simulink model "exo2_Part1_y"  (R2020b)
settings: Solver=VariableStepAuto  StartTime=0.0  StopTime=30  RelTol=1e-3
undefined symbols (not defined in the file or in its folder): fdesignblkfcn, gcbh
libraries: dspfdesign x4, vrlib x1
settings Model: Creator=aayush  LastModifiedBy=YNS
settings DebuggingCC: UnconnectedInputMsg=none  UnconnectedOutputMsg=none  UnconnectedLineMsg=none
settings ModelReferenceCC: EnableRefExpFcnMdlSchedulingChecks=off

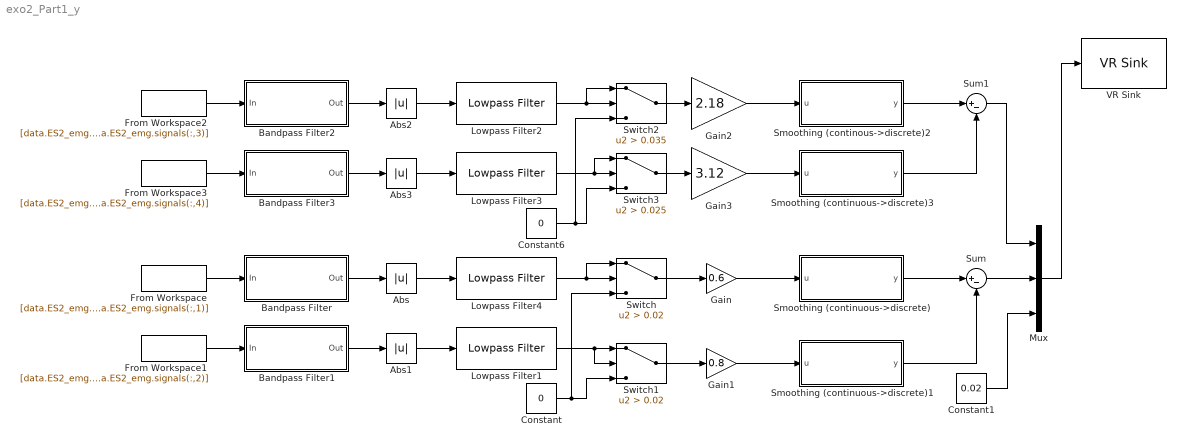
== system exo2_Part1_y ==
  Abs{,1..3} (4 alike) : Abs
  Bandpass Filter : Subsystem  DialogController=fdesignblkfcn  InitFcn=fdesignblkfcn(gcbh, {'InitFcn'});  mask(Bandpass Filter){}
      mask help: Design a bandpass filter
      settings: CopyFcn=fdesignblkfcn(gcbh, {'CopyFcn'});
      mask Help: helpview(mapfilelocation('dsp'), 'dspbandpassfilter');
      mask Display: disp('Bandpass');
  Bandpass Filter1 : Subsystem  DialogController=fdesignblkfcn  InitFcn=fdesignblkfcn(gcbh, {'InitFcn'});  mask(Bandpass Filter){}
      mask help: Design a bandpass filter
      settings: CopyFcn=fdesignblkfcn(gcbh, {'CopyFcn'});
      mask Help: helpview(mapfilelocation('dsp'), 'dspbandpassfilter');
      mask Display: disp('Bandpass');
  Bandpass Filter2 : Subsystem  DialogController=fdesignblkfcn  InitFcn=fdesignblkfcn(gcbh, {'InitFcn'});  mask(Bandpass Filter){}
      mask help: Design a bandpass filter
      settings: CopyFcn=fdesignblkfcn(gcbh, {'CopyFcn'});
      mask Help: helpview(mapfilelocation('dsp'), 'dspbandpassfilter');
      mask Display: disp('Bandpass');
  Bandpass Filter3 : Subsystem  DialogController=fdesignblkfcn  InitFcn=fdesignblkfcn(gcbh, {'InitFcn'});  mask(Bandpass Filter){}
      mask help: Design a bandpass filter
      settings: CopyFcn=fdesignblkfcn(gcbh, {'CopyFcn'});
      mask Help: helpview(mapfilelocation('dsp'), 'dspbandpassfilter');
      mask Display: disp('Bandpass');
  Constant : Constant  Value=0
  Constant1 : Constant  Value=0.02
  Constant6 : Constant  Value=0
  From Workspace : FromWorkspace  VariableName=[data.ES2_emg.time,data.ES2_emg.signals(:,1)]  SampleTime=1/3000
  From Workspace1 : FromWorkspace  VariableName=[data.ES2_emg.time,data.ES2_emg.signals(:,2)]  SampleTime=1/3000
  From Workspace2 : FromWorkspace  VariableName=[data.ES2_emg.time,data.ES2_emg.signals(:,3)]  SampleTime=1/3000
  From Workspace3 : FromWorkspace  VariableName=[data.ES2_emg.time,data.ES2_emg.signals(:,4)]  SampleTime=1/3000
  Gain : Gain  Gain=0.6
  Gain1 : Gain  Gain=0.8
  Gain2 : Gain  Gain=2.18
  Gain3 : Gain  Gain=3.12
  Lowpass Filter{1..4} (4 alike) : dspfdesign/Lowpass Filter  FilterType=FIR  DesignForMinimumOrder=on  FilterOrder=50  PassbandFrequency=3  StopbandFrequency=6  PassbandRipple=0.1  StopbandAttenuation=80  InheritSampleRate=off  SampleRate=1000  SimulateUsing=Interpreted execution  roundingMode=Floor  coeffsDataTypeStr=fixdt(1,16)
  Mux : Mux  Inputs=3
  Smoothing (continous->discrete)2 : Subsystem  mask(Smoothing (continuous->discrete)){tsSmoothing=0.35, smoothing0=0}
      mask prompts: tsSmoothing "physmod:simscape:couplers:SimscapeNetworkCouplersLib:SmoothingTimeConstants_MP"; smoothing0 "physmod:simscape:couplers:SimscapeNetworkCouplersLib:InitialOutput_MP"
      mask help: physmod:simscape:couplers:SimscapeNetworkCouplersLib:Smoothingcontinuousdiscrete_MD
      mask Help: web([docroot '/physmod/simscape/ref/networkcouplersmoothingcontinuousdiscrete.html'])
  Smoothing (continuous->discrete) : Subsystem  mask(Smoothing (continuous->discrete)){tsSmoothing=0.35, smoothing0=0}
      mask prompts: tsSmoothing "physmod:simscape:couplers:SimscapeNetworkCouplersLib:SmoothingTimeConstants_MP"; smoothing0 "physmod:simscape:couplers:SimscapeNetworkCouplersLib:InitialOutput_MP"
      mask help: physmod:simscape:couplers:SimscapeNetworkCouplersLib:Smoothingcontinuousdiscrete_MD
      mask Help: web([docroot '/physmod/simscape/ref/networkcouplersmoothingcontinuousdiscrete.html'])
  Smoothing (continuous->discrete)1 : Subsystem  mask(Smoothing (continuous->discrete)){tsSmoothing=0.35, smoothing0=0}
      mask prompts: tsSmoothing "physmod:simscape:couplers:SimscapeNetworkCouplersLib:SmoothingTimeConstants_MP"; smoothing0 "physmod:simscape:couplers:SimscapeNetworkCouplersLib:InitialOutput_MP"
      mask help: physmod:simscape:couplers:SimscapeNetworkCouplersLib:Smoothingcontinuousdiscrete_MD
      mask Help: web([docroot '/physmod/simscape/ref/networkcouplersmoothingcontinuousdiscrete.html'])
  Smoothing (continuous->discrete)3 : Subsystem  mask(Smoothing (continuous->discrete)){tsSmoothing=0.35, smoothing0=0}
      mask prompts: tsSmoothing "physmod:simscape:couplers:SimscapeNetworkCouplersLib:SmoothingTimeConstants_MP"; smoothing0 "physmod:simscape:couplers:SimscapeNetworkCouplersLib:InitialOutput_MP"
      mask help: physmod:simscape:couplers:SimscapeNetworkCouplersLib:Smoothingcontinuousdiscrete_MD
      mask Help: web([docroot '/physmod/simscape/ref/networkcouplersmoothingcontinuousdiscrete.html'])
  Sum : Sum  Inputs=|+-
  Sum1 : Sum  Inputs=|+-
  Switch : Switch  Criteria=u2 > Threshold  Threshold=0.02
  Switch1 : Switch  Criteria=u2 > Threshold  Threshold=0.02
  Switch2 : Switch  Criteria=u2 > Threshold  Threshold=0.035
  Switch3 : Switch  Criteria=u2 > Threshold  Threshold=0.025
  VR Sink : vrlib/VR Sink  InstantiateOnLoad=on  SampleTime=0.1  ViewEnable=on  RemoteChange=off  RemoteView=off  FieldsWritten=cursor.translation.3.1.1.double  WorldFileName=8_palline_color.wrl  AutoView=off  VideoDimensions=[]  AllowVariableSize=off  FigureProperties="{'Position', 'Name', 'Viewpoint', 'CameraBound', 'CameraDirection', 'CameraPosition', 'CameraUpVector', 'ZoomFactor', 'Antialiasing', 'Headlight', 'Lighting', 'NavPanel', 'Sound', 'StatusBar', 'Stereo3D', 'Stereo3DCameraOffset', 'Stereo3DHIT', 'ToolBar', 'Textures', 'Transparency', 'Triad', 'Wireframe', 'NavZones', 'NavMode', 'NavSpeed', 'CaptureFileFormat', 'CaptureFileName', 'Record2DCompressMethod', 'Record2DCompressQuality', 'Record2D', 'Record2DFileName', 'Record2DFPS'; [5.0000000000000000e+00   9.2000000000000000e+01   5.7600000000000000e+02   3.5000000000000000e+02], '', '_untitled_1', 'on', [0.0000000000000000e+00   0.0000000000000000e+00  -1.0000000000000000e+00], [0.0000000000000000e+00   0.0000000000000000e+00   0.0000000000000000e+00], [0.0000000000000000e+00   1.0000000000000000e+00   0.0000000000000000e+00], [1.0000000000000000e+00], 'on', 'on', 'on', 'halfbar', 'on', 'on', 'off', [1.0000000149011612e-01], [0.0000000000000000e+00], 'on', 'on', 'on', 'none', 'off', 'off', 'walk', 'normal', 'tif', '%f_anim_%n.tif', 'auto', [7.5000000000000000e+01], 'off', '%f_anim_%n.avi', 'auto'}"
  wires:
  Constant6/1 -> Switch2/3, Switch3/3
  Bandpass Filter2/1(Out) -> Abs2/1
  From Workspace/1 -> Bandpass Filter/1(In)
  From Workspace2/1 -> Bandpass Filter2/1(In)
  From Workspace3/1 -> Bandpass Filter3/1(In)
  Bandpass Filter/1(Out) -> Abs/1
  From Workspace1/1 -> Bandpass Filter1/1(In)
  Bandpass Filter3/1(Out) -> Abs3/1
  Bandpass Filter1/1(Out) -> Abs1/1
  Abs/1 -> Lowpass Filter4/1
  Abs2/1 -> Lowpass Filter2/1
  Abs3/1 -> Lowpass Filter3/1
  Abs1/1 -> Lowpass Filter1/1
  Smoothing (continuous->discrete)1/1(y) -> Sum/2
  Lowpass Filter2/1 -> Switch2/1, Switch2/2
  Smoothing (continous->discrete)2/1(y) -> Sum1/1
  Lowpass Filter3/1 -> Switch3/1, Switch3/2
  Lowpass Filter4/1 -> Switch/1, Switch/2
  Lowpass Filter1/1 -> Switch1/1, Switch1/2
  Gain1/1 -> Smoothing (continuous->discrete)1/1(u)
  Constant/1 -> Switch/3, Switch1/3
  Switch2/1 -> Gain2/1
  Switch3/1 -> Gain3/1
  Gain2/1 -> Smoothing (continous->discrete)2/1(u)
  Switch/1 -> Gain/1
  Constant1/1 -> Mux/3
  Switch1/1 -> Gain1/1
  Gain3/1 -> Smoothing (continuous->discrete)3/1(u)
  Gain/1 -> Smoothing (continuous->discrete)/1(u)
  Smoothing (continuous->discrete)3/1(y) -> Sum1/2
  Smoothing (continuous->discrete)/1(y) -> Sum/1
  Sum1/1 -> Mux/1
  Sum/1 -> Mux/2
  Mux/1 -> VR Sink/1

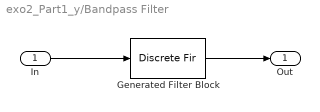
== system exo2_Part1_y/Bandpass Filter ==
  In : Inport
  Generated Filter Block : DiscreteFir  Tag=BlockMethodSubSystem  Coefficients=[0.0247784165301608433 0.00982645761123041028 -0.076956364309928485 -0.00574234407939242311 -0.0280411528162793217 -0.00804608705322140162 -0.0118695570715928369 -0.00997698951682126148 -0.0032900682882155835 -0.0123964456094048502 0.00352600878115876329 -0.0139189700142880405 0.00905023941727317073 -0.0130997642055635105 0.0124656128815527987 -0.00909287544946293935 0.0131317697099942975 -0.00207947540041804888 0.0111769210630364487 0.00659009778413368903 0.00765273613394504455 0.0147232835745342554 0.00427867752512019368 0.0199633122366019398 0.00267711132018813233 0.0203811397583988814 0.0037418940950067715 0.0149169811807585064 0.00742876303379174253 0.00413015922899517742 0.0123258049521986213 -0.00967745920215465696 0.015760250203825283 -0.0236422789640416652 0.0148621759121691233 -0.0338874815186639144 0.00685197471547598861 -0.0377812878977663025 -0.00958300552505572667 -0.0336540649346103726 -0.0340410723239205834 -0.0220502805385552648 -0.063942206809497748 -0.00527010472050306374 -0.0951066582635559377 0.0128546225834283885 -0.12245473858081414 0.0280548282114237782 -0.141172435722598355 0.0367254315914400456 0.852170468203800047 0.0367254315914400456 -0.141172435722598355 0.0280548282114237782 -0.12245473858081414 0.0128546225834283885 -0.0951066582635559377 -0.00527010472050306374 -0.063942206809497748 -0.0220502805385552648 -0.0340410723239205834 -0.0336540649346103726 -0.00958300552505572667 -0.0377812878977663025 0.00685197471547598861 -0.0338874815186639144 0.0148621759121691233 -0.0236422789640416652 0.015760250203825283 -0.00967745920215465696 0.0123258049521986213 0.00413015922899517742 0.00742876303379174253 0.0149169811807585064 0.0037418940950067715 0.0203811397583988814 0.00267711132018813233 0.0199633122366019398 0.00427867752512019368 0.0147232835745342554 0.00765273613394504455 0.00659009778413368903 0.0111769210630364487 -0.00207947540041804888 0.0131317697099942975 -0.00909287544946293935 0.0124656128815527987 -0.0130997642055635105 0.00905023941727317073 -0.0139189700142880405 0.00352600878115876329 -0.0123964456094048502 -0.0032900682882155835 -0.00997698951682126148 -0.0118695570715928369 -0.00804608705322140162 -0.0280411528162793217 -0.00574234407939242311 -0.076956364309928485 0.00982645761123041028 0.0247784165301608433]  InputProcessing=Columns as channels (frame based)
  Out : Outport  VectorParamsAs1DForOutWhenUnconnected=off
  wires:
  In/1 -> Generated Filter Block/1
  Generated Filter Block/1 -> Out/1

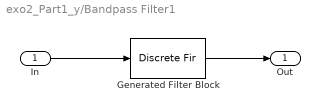
== system exo2_Part1_y/Bandpass Filter1 ==
  In : Inport
  Generated Filter Block : DiscreteFir  Tag=BlockMethodSubSystem  Coefficients=[0.0247784165301608433 0.00982645761123041028 -0.076956364309928485 -0.00574234407939242311 -0.0280411528162793217 -0.00804608705322140162 -0.0118695570715928369 -0.00997698951682126148 -0.0032900682882155835 -0.0123964456094048502 0.00352600878115876329 -0.0139189700142880405 0.00905023941727317073 -0.0130997642055635105 0.0124656128815527987 -0.00909287544946293935 0.0131317697099942975 -0.00207947540041804888 0.0111769210630364487 0.00659009778413368903 0.00765273613394504455 0.0147232835745342554 0.00427867752512019368 0.0199633122366019398 0.00267711132018813233 0.0203811397583988814 0.0037418940950067715 0.0149169811807585064 0.00742876303379174253 0.00413015922899517742 0.0123258049521986213 -0.00967745920215465696 0.015760250203825283 -0.0236422789640416652 0.0148621759121691233 -0.0338874815186639144 0.00685197471547598861 -0.0377812878977663025 -0.00958300552505572667 -0.0336540649346103726 -0.0340410723239205834 -0.0220502805385552648 -0.063942206809497748 -0.00527010472050306374 -0.0951066582635559377 0.0128546225834283885 -0.12245473858081414 0.0280548282114237782 -0.141172435722598355 0.0367254315914400456 0.852170468203800047 0.0367254315914400456 -0.141172435722598355 0.0280548282114237782 -0.12245473858081414 0.0128546225834283885 -0.0951066582635559377 -0.00527010472050306374 -0.063942206809497748 -0.0220502805385552648 -0.0340410723239205834 -0.0336540649346103726 -0.00958300552505572667 -0.0377812878977663025 0.00685197471547598861 -0.0338874815186639144 0.0148621759121691233 -0.0236422789640416652 0.015760250203825283 -0.00967745920215465696 0.0123258049521986213 0.00413015922899517742 0.00742876303379174253 0.0149169811807585064 0.0037418940950067715 0.0203811397583988814 0.00267711132018813233 0.0199633122366019398 0.00427867752512019368 0.0147232835745342554 0.00765273613394504455 0.00659009778413368903 0.0111769210630364487 -0.00207947540041804888 0.0131317697099942975 -0.00909287544946293935 0.0124656128815527987 -0.0130997642055635105 0.00905023941727317073 -0.0139189700142880405 0.00352600878115876329 -0.0123964456094048502 -0.0032900682882155835 -0.00997698951682126148 -0.0118695570715928369 -0.00804608705322140162 -0.0280411528162793217 -0.00574234407939242311 -0.076956364309928485 0.00982645761123041028 0.0247784165301608433]  InputProcessing=Columns as channels (frame based)
  Out : Outport  VectorParamsAs1DForOutWhenUnconnected=off
  wires:
  In/1 -> Generated Filter Block/1
  Generated Filter Block/1 -> Out/1

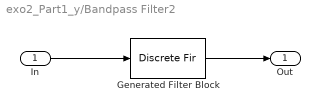
== system exo2_Part1_y/Bandpass Filter2 ==
  In : Inport
  Generated Filter Block : DiscreteFir  Tag=BlockMethodSubSystem  Coefficients=[0.0247784165301608433 0.00982645761123041028 -0.076956364309928485 -0.00574234407939242311 -0.0280411528162793217 -0.00804608705322140162 -0.0118695570715928369 -0.00997698951682126148 -0.0032900682882155835 -0.0123964456094048502 0.00352600878115876329 -0.0139189700142880405 0.00905023941727317073 -0.0130997642055635105 0.0124656128815527987 -0.00909287544946293935 0.0131317697099942975 -0.00207947540041804888 0.0111769210630364487 0.00659009778413368903 0.00765273613394504455 0.0147232835745342554 0.00427867752512019368 0.0199633122366019398 0.00267711132018813233 0.0203811397583988814 0.0037418940950067715 0.0149169811807585064 0.00742876303379174253 0.00413015922899517742 0.0123258049521986213 -0.00967745920215465696 0.015760250203825283 -0.0236422789640416652 0.0148621759121691233 -0.0338874815186639144 0.00685197471547598861 -0.0377812878977663025 -0.00958300552505572667 -0.0336540649346103726 -0.0340410723239205834 -0.0220502805385552648 -0.063942206809497748 -0.00527010472050306374 -0.0951066582635559377 0.0128546225834283885 -0.12245473858081414 0.0280548282114237782 -0.141172435722598355 0.0367254315914400456 0.852170468203800047 0.0367254315914400456 -0.141172435722598355 0.0280548282114237782 -0.12245473858081414 0.0128546225834283885 -0.0951066582635559377 -0.00527010472050306374 -0.063942206809497748 -0.0220502805385552648 -0.0340410723239205834 -0.0336540649346103726 -0.00958300552505572667 -0.0377812878977663025 0.00685197471547598861 -0.0338874815186639144 0.0148621759121691233 -0.0236422789640416652 0.015760250203825283 -0.00967745920215465696 0.0123258049521986213 0.00413015922899517742 0.00742876303379174253 0.0149169811807585064 0.0037418940950067715 0.0203811397583988814 0.00267711132018813233 0.0199633122366019398 0.00427867752512019368 0.0147232835745342554 0.00765273613394504455 0.00659009778413368903 0.0111769210630364487 -0.00207947540041804888 0.0131317697099942975 -0.00909287544946293935 0.0124656128815527987 -0.0130997642055635105 0.00905023941727317073 -0.0139189700142880405 0.00352600878115876329 -0.0123964456094048502 -0.0032900682882155835 -0.00997698951682126148 -0.0118695570715928369 -0.00804608705322140162 -0.0280411528162793217 -0.00574234407939242311 -0.076956364309928485 0.00982645761123041028 0.0247784165301608433]  InputProcessing=Columns as channels (frame based)
  Out : Outport  VectorParamsAs1DForOutWhenUnconnected=off
  wires:
  In/1 -> Generated Filter Block/1
  Generated Filter Block/1 -> Out/1

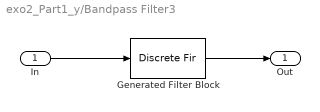
== system exo2_Part1_y/Bandpass Filter3 ==
  In : Inport
  Generated Filter Block : DiscreteFir  Tag=BlockMethodSubSystem  Coefficients=[0.0247784165301608433 0.00982645761123041028 -0.076956364309928485 -0.00574234407939242311 -0.0280411528162793217 -0.00804608705322140162 -0.0118695570715928369 -0.00997698951682126148 -0.0032900682882155835 -0.0123964456094048502 0.00352600878115876329 -0.0139189700142880405 0.00905023941727317073 -0.0130997642055635105 0.0124656128815527987 -0.00909287544946293935 0.0131317697099942975 -0.00207947540041804888 0.0111769210630364487 0.00659009778413368903 0.00765273613394504455 0.0147232835745342554 0.00427867752512019368 0.0199633122366019398 0.00267711132018813233 0.0203811397583988814 0.0037418940950067715 0.0149169811807585064 0.00742876303379174253 0.00413015922899517742 0.0123258049521986213 -0.00967745920215465696 0.015760250203825283 -0.0236422789640416652 0.0148621759121691233 -0.0338874815186639144 0.00685197471547598861 -0.0377812878977663025 -0.00958300552505572667 -0.0336540649346103726 -0.0340410723239205834 -0.0220502805385552648 -0.063942206809497748 -0.00527010472050306374 -0.0951066582635559377 0.0128546225834283885 -0.12245473858081414 0.0280548282114237782 -0.141172435722598355 0.0367254315914400456 0.852170468203800047 0.0367254315914400456 -0.141172435722598355 0.0280548282114237782 -0.12245473858081414 0.0128546225834283885 -0.0951066582635559377 -0.00527010472050306374 -0.063942206809497748 -0.0220502805385552648 -0.0340410723239205834 -0.0336540649346103726 -0.00958300552505572667 -0.0377812878977663025 0.00685197471547598861 -0.0338874815186639144 0.0148621759121691233 -0.0236422789640416652 0.015760250203825283 -0.00967745920215465696 0.0123258049521986213 0.00413015922899517742 0.00742876303379174253 0.0149169811807585064 0.0037418940950067715 0.0203811397583988814 0.00267711132018813233 0.0199633122366019398 0.00427867752512019368 0.0147232835745342554 0.00765273613394504455 0.00659009778413368903 0.0111769210630364487 -0.00207947540041804888 0.0131317697099942975 -0.00909287544946293935 0.0124656128815527987 -0.0130997642055635105 0.00905023941727317073 -0.0139189700142880405 0.00352600878115876329 -0.0123964456094048502 -0.0032900682882155835 -0.00997698951682126148 -0.0118695570715928369 -0.00804608705322140162 -0.0280411528162793217 -0.00574234407939242311 -0.076956364309928485 0.00982645761123041028 0.0247784165301608433]  InputProcessing=Columns as channels (frame based)
  Out : Outport  VectorParamsAs1DForOutWhenUnconnected=off
  wires:
  In/1 -> Generated Filter Block/1
  Generated Filter Block/1 -> Out/1

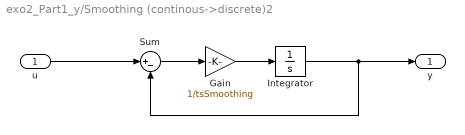
== system exo2_Part1_y/Smoothing (continous->discrete)2 ==
  u : Inport
  Gain : Gain  Gain=1/tsSmoothing
  Integrator : Integrator  InitialCondition=smoothing0
  Sum : Sum  Inputs=|+-
  y : Outport
  wires:
  u/1 -> Sum/1
  Integrator/1 -> Sum/2, y/1
  Gain/1 -> Integrator/1
  Sum/1 -> Gain/1

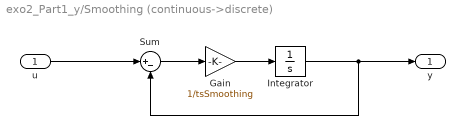
== system exo2_Part1_y/Smoothing (continuous->discrete) ==
  u : Inport
  Gain : Gain  Gain=1/tsSmoothing
  Integrator : Integrator  InitialCondition=smoothing0
  Sum : Sum  Inputs=|+-
  y : Outport
  wires:
  u/1 -> Sum/1
  Integrator/1 -> Sum/2, y/1
  Gain/1 -> Integrator/1
  Sum/1 -> Gain/1

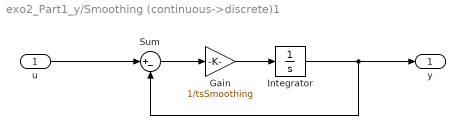
== system exo2_Part1_y/Smoothing (continuous->discrete)1 ==
  u : Inport
  Gain : Gain  Gain=1/tsSmoothing
  Integrator : Integrator  InitialCondition=smoothing0
  Sum : Sum  Inputs=|+-
  y : Outport
  wires:
  u/1 -> Sum/1
  Integrator/1 -> Sum/2, y/1
  Gain/1 -> Integrator/1
  Sum/1 -> Gain/1

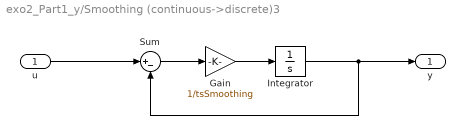
== system exo2_Part1_y/Smoothing (continuous->discrete)3 ==
  u : Inport
  Gain : Gain  Gain=1/tsSmoothing
  Integrator : Integrator  InitialCondition=smoothing0
  Sum : Sum  Inputs=|+-
  y : Outport
  wires:
  u/1 -> Sum/1
  Integrator/1 -> Sum/2, y/1
  Gain/1 -> Integrator/1
  Sum/1 -> Gain/1
